simulink model "finalpro"  (R2021a)
settings: Solver=FixedStepAuto  StartTime=0.0  StopTime=25  FixedStep=0.001  RelTol=1e-3
libraries: neural x8, pid_lib x4, fuzblock x1
settings Model: Creator=User  LastModifiedBy=User

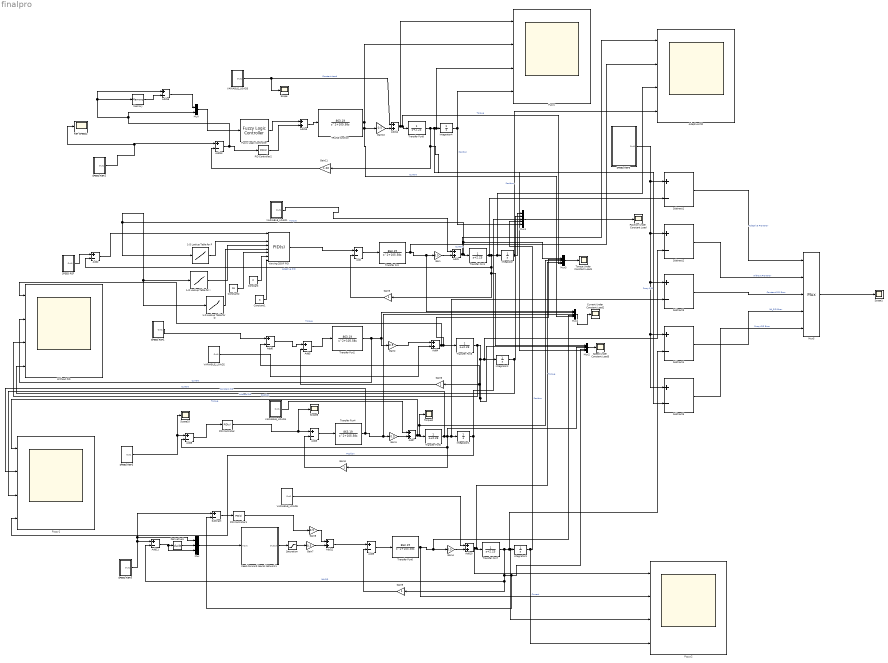
== system finalpro ==
  1-D Lookup Table for D : Lookup_n-D  NumberOfTableDimensions=1  BreakpointsForDimension1=[-5, -4.5, -4, -3.5, -3, -2.5, -2, -1.5, -1, -0.5, 0, 0.5, 1, 1.5, 2, 2.5, 3, 3.5, 4, 4.5, 5, 5.5, 6, 6.5, 7, 7.5, 8, 8.5, 9, 9.5, 10]  Table=[0.1, 0.1, 0.1, 0.1, 0.1, 0.1, 0.1, 0.1, 0.1, 0.1, 0.1, 0.1, 0.1, 0.1, 0.1, 0.1, 0.1, 0.1, 0.1, 0.1, 0.1, 0.1, 0.1, 0.1, 0.1, 0.1, 0.1, 0.1, 0.1, 0.1, 0.1]  InterpMethod=Linear Lagrange  InternalRulePriority=Speed  RndMeth=Simplest  InputSameDT=on
  1-D Lookup Table for I : Lookup_n-D  NumberOfTableDimensions=1  BreakpointsForDimension1=[-5, -4.5, -4, -3.5, -3, -2.5, -2, -1.5, -1, -0.5, 0, 0.5, 1, 1.5, 2, 2.5, 3, 3.5, 4, 4.5, 5, 5.5, 6, 6.5, 7, 7.5, 8, 8.5, 9, 9.5, 10]  Table=[2.0, 2.0, 2.0, 2.0, 2.0, 0.1, 0.1, 0.1, 2.0, 0.5, 0.5, 0.5, 0.5, 0.5, 0.5, 2.5, 2.5, 2.5, 2.0, 2.0, 2.0, 2.0, 0.5, 0.5, 0.5, 2.0, 2.0, 2.0, 2.0, 2.0, 2.0]  InternalRulePriority=Speed  RndMeth=Simplest  InputSameDT=on
  1-D Lookup Table for P : Lookup_n-D  NumberOfTableDimensions=1  BreakpointsForDimension1=[-5, -4.5, -4, -3.5, -3, -2.5, -2, -1.5, -1, -0.5, 0, 0.5, 1, 1.5, 2, 2.5, 3, 3.5, 4, 4.5, 5, 5.5, 6, 6.5, 7, 7.5, 8, 8.5, 9, 9.5, 10]  Table=[2.0, 2.0, 0.5, 0.05, 0.05, 0.5, 0.1, 1, 1.5, 1.5, 1.5, 1.5, 2.0, 2.0, 2.5, .05, .5, .5, 2.0, 2.0, 2.0, 2.0, 0.5, 0.5, 0.5, 2.0, 2.0, 2.0, 2.0, 2.0, 2.0]  InterpMethod=Linear Lagrange  InternalRulePriority=Speed  RndMeth=Simplest  InputSameDT=on
  Adaptive PID : Scope  NumInputPorts=4
  Add{,2..3,5..6,8..9,11,13,16} (10 alike) : Sum  Inputs=+-
  Add{1,4,7,10,12,14..15} (7 alike) : Sum
  Constant : Constant  Value=2
  Constant1 : Constant  Value=3
  Constant2 : Constant  Value=15
  Current Under Constant Load2 : Scope
  Derivative1 : Derivative
  Feed-Forward Neural Network1 : Subsystem
      mask help: Feed-Forward Neural Network
      mask Display: e = 0.06;c1 = [120 150 230]/255;c2 = ([120 150 230]+0)/383;c3 = ([120 150 230]+128)/383;patch([0 1 1 0],[0 0 1 1],c1);patch([0 1 1 1-e 1-e 0+e],[0 0 1 1-e 0+e 0+e],c2);patch([0 0 1 1-e 0+e 0+e],[0 1 1 1-e 1-e 0+e],c3);plot([0 1 1 0 0],[0 0 1 1 0]);fprintf('NNET');port_label('input',1,' Input');port_label('output',1,'Output ');
  Fuzzy : Scope  NumInputPorts=4
  Fuzzy Logic Controller : fuzblock/Fuzzy Logic  Controller  FIS='DCMotorFLC.fis'  OutputSampleNumber=101  DataType=double  FuzzifiedInputs=off  RuleFiringStrengths=off  RuleOutputs=off  AggregatedOutputs=off  SimulateUsing=Interpreted execution  OutOfRangeInputValueMessage=warning  NoRuleFiredMessage=warning  EmptyOutputFuzzySetMessage=warning
  Fuzzy1 : Scope  NumInputPorts=4
  Fuzzy2 : Scope  NumInputPorts=4
  Gain{,1..2,4,7..8,10} (7 alike) : Gain  Gain=0.5
  Gain11 : Gain  Gain=1.02
  Gain{3,5..6,9} (4 alike) : Gain
  Integrator{,1..4} (5 alike) : Integrator
  MUX : Mux  Inputs=2
  Memory : Memory
  Mux : Mux  Inputs=3
  Mux{1..5} (5 alike) : Mux  Inputs=5
  PID Controller : pid_lib/PID Controller  Controller=PID  Form=Parallel  TimeDomain=Continuous-time  UseExternalTs=off  SampleTime=-1  IntegratorMethod=Forward Euler  FilterMethod=Forward Euler  ControllerParametersSource=internal  P=2  I=2.2  D=0.8  UseFilter=on  N=358.799773599194  TunerSelectOption=Transfer Function Based (PID Tuner App)  InitialConditionSource=internal  InitialConditionForIntegrator=0  InitialConditionForFilter=0  DifferentiatorICPrevScaledInput=0  ExternalReset=none  TrackingMode=off  Kt=1  LimitOutput=off  SatLimitsSource=internal  UpperSaturationLimit=inf  LowerSaturationLimit=-inf  LinearizeAsGain=on  AntiWindupMode=none  Kb=1  POutMin=[]  POutMax=[]  IOutMin=[]  IOutMax=[]  DOutMin=[]  DOutMax=[]  NOutMin=[]  NOutMax=[]  SumOutMin=[]  SumOutMax=[]  SaturationOutMin=[]  SaturationOutMax=[]  PParamMin=[]  PParamMax=[]  IParamMin=[]  IParamMax=[]  DParamMin=[]  DParamMax=[]  NParamMin=[]  NParamMax=[]  KbParamMin=[]  KbParamMax=[]  KtParamMin=[]  KtParamMax=[]  KbOutMin=[]  KbOutMax=[]  KtOutMin=[]  KtOutMax=[]  IntegratorOutMin=[]  IntegratorOutMax=[]  FilterOutMin=[]  FilterOutMax=[]  SumI1OutMin=[]  SumI1OutMax=[]  SumI2OutMin=[]  SumI2OutMax=[]  SumI3OutMin=[]  SumI3OutMax=[]  SumI4OutMin=[]  SumI4OutMax=[]  SumDOutMin=[]  SumDOutMax=[]  DifferentiatorOutMin=[]  DifferentiatorOutMax=[]  FilterDiffOutCoefMin=[]  FilterDiffOutCoefMax=[]  ReciprocalOutMin=[]  ReciprocalOutMax=[]  SumDenOutMin=[]  SumDenOutMax=[]  SumNumOutMin=[]  SumNumOutMax=[]  DivideOutMin=[]  DivideOutMax=[]  UdiffTsProdOutMin=[]  UdiffTsProdOutMax=[]  NTsProdOutMin=[]  NTsProdOutMax=[]  UintegralTsProdOutMin=[]  UintegralTsProdOutMax=[]  UngainTsProdOutMin=[]  UngainTsProdOutMax=[]  IntegratorContinuousStateAttributes=''  IntegratorStateMustResolveToSignalObject=off  IntegratorRTWStateStorageClass=Auto  FilterContinuousStateAttributes=''  FilterStateMustResolveToSignalObject=off  FilterRTWStateStorageClass=Auto  ParallelPVariant=InternalParameters  IdealPVariant=Disabled  IVariant=InternalParameters  DVariant=InternalParameters  IntegratorVariant=Continuous  SatVariant=Disabled  AWVariant=Passthrough  PCopyVariant=Disabled  TRVariant=Disabled  FdbkBlocksVariant=Forward  IdealPFdbkVariant=Disabled  SatFdbkVariant=Disabled  DerivativeFilterVariant=ContFilter  NVariant=InternalParameters  NCopyVariant=Disabled  FilterICVariant=InternalICsFilter  IntegratorICVariant=InternalICs  ExternalResetVariant=Disabled  TRSumVariant=Passthrough  SumFdbkVariant=Disabled  SumVariant=Sum_PID  TsampFilterVariant=InternalTs  TsampNgainVariant=Passthrough  TsampIntegralVariant=Passthrough  ExternalSaturationOutDataTypeStr=Inherit: Same as second input
  PID Controller1 : pid_lib/PID Controller  Controller=PID  Form=Parallel  TimeDomain=Continuous-time  UseExternalTs=off  SampleTime=-1  IntegratorMethod=Forward Euler  FilterMethod=Forward Euler  ControllerParametersSource=internal  P=2  I=2.2  D=0.8  UseFilter=on  N=358.799773599194  TunerSelectOption=Transfer Function Based (PID Tuner App)  InitialConditionSource=internal  InitialConditionForIntegrator=0  InitialConditionForFilter=0  DifferentiatorICPrevScaledInput=0  ExternalReset=none  TrackingMode=off  Kt=1  LimitOutput=off  SatLimitsSource=internal  UpperSaturationLimit=inf  LowerSaturationLimit=-inf  LinearizeAsGain=on  AntiWindupMode=none  Kb=1  POutMin=[]  POutMax=[]  IOutMin=[]  IOutMax=[]  DOutMin=[]  DOutMax=[]  NOutMin=[]  NOutMax=[]  SumOutMin=[]  SumOutMax=[]  SaturationOutMin=[]  SaturationOutMax=[]  PParamMin=[]  PParamMax=[]  IParamMin=[]  IParamMax=[]  DParamMin=[]  DParamMax=[]  NParamMin=[]  NParamMax=[]  KbParamMin=[]  KbParamMax=[]  KtParamMin=[]  KtParamMax=[]  KbOutMin=[]  KbOutMax=[]  KtOutMin=[]  KtOutMax=[]  IntegratorOutMin=[]  IntegratorOutMax=[]  FilterOutMin=[]  FilterOutMax=[]  SumI1OutMin=[]  SumI1OutMax=[]  SumI2OutMin=[]  SumI2OutMax=[]  SumI3OutMin=[]  SumI3OutMax=[]  SumI4OutMin=[]  SumI4OutMax=[]  SumDOutMin=[]  SumDOutMax=[]  DifferentiatorOutMin=[]  DifferentiatorOutMax=[]  FilterDiffOutCoefMin=[]  FilterDiffOutCoefMax=[]  ReciprocalOutMin=[]  ReciprocalOutMax=[]  SumDenOutMin=[]  SumDenOutMax=[]  SumNumOutMin=[]  SumNumOutMax=[]  DivideOutMin=[]  DivideOutMax=[]  UdiffTsProdOutMin=[]  UdiffTsProdOutMax=[]  NTsProdOutMin=[]  NTsProdOutMax=[]  UintegralTsProdOutMin=[]  UintegralTsProdOutMax=[]  UngainTsProdOutMin=[]  UngainTsProdOutMax=[]  IntegratorContinuousStateAttributes=''  IntegratorStateMustResolveToSignalObject=off  IntegratorRTWStateStorageClass=Auto  FilterContinuousStateAttributes=''  FilterStateMustResolveToSignalObject=off  FilterRTWStateStorageClass=Auto  ParallelPVariant=InternalParameters  IdealPVariant=Disabled  IVariant=InternalParameters  DVariant=InternalParameters  IntegratorVariant=Continuous  SatVariant=Disabled  AWVariant=Passthrough  PCopyVariant=Disabled  TRVariant=Disabled  FdbkBlocksVariant=Forward  IdealPFdbkVariant=Disabled  SatFdbkVariant=Disabled  DerivativeFilterVariant=ContFilter  NVariant=InternalParameters  NCopyVariant=Disabled  FilterICVariant=InternalICsFilter  IntegratorICVariant=InternalICs  ExternalResetVariant=Disabled  TRSumVariant=Passthrough  SumFdbkVariant=Disabled  SumVariant=Sum_PID  TsampFilterVariant=InternalTs  TsampNgainVariant=Passthrough  TsampIntegralVariant=Passthrough  ExternalSaturationOutDataTypeStr=Inherit: Same as second input
  PID Controller2 : pid_lib/PID Controller  Controller=PID  Form=Parallel  TimeDomain=Continuous-time  UseExternalTs=off  SampleTime=-1  IntegratorMethod=Forward Euler  FilterMethod=Forward Euler  ControllerParametersSource=internal  P=1.8  I=0.6  D=0.5  UseFilter=on  N=100  TunerSelectOption=Transfer Function Based (PID Tuner App)  InitialConditionSource=internal  InitialConditionForIntegrator=0  InitialConditionForFilter=0  DifferentiatorICPrevScaledInput=0  ExternalReset=none  TrackingMode=off  Kt=1  LimitOutput=off  SatLimitsSource=internal  UpperSaturationLimit=inf  LowerSaturationLimit=-inf  LinearizeAsGain=on  AntiWindupMode=none  Kb=1  POutMin=[]  POutMax=[]  IOutMin=[]  IOutMax=[]  DOutMin=[]  DOutMax=[]  NOutMin=[]  NOutMax=[]  SumOutMin=[]  SumOutMax=[]  SaturationOutMin=[]  SaturationOutMax=[]  PParamMin=[]  PParamMax=[]  IParamMin=[]  IParamMax=[]  DParamMin=[]  DParamMax=[]  NParamMin=[]  NParamMax=[]  KbParamMin=[]  KbParamMax=[]  KtParamMin=[]  KtParamMax=[]  KbOutMin=[]  KbOutMax=[]  KtOutMin=[]  KtOutMax=[]  IntegratorOutMin=[]  IntegratorOutMax=[]  FilterOutMin=[]  FilterOutMax=[]  SumI1OutMin=[]  SumI1OutMax=[]  SumI2OutMin=[]  SumI2OutMax=[]  SumI3OutMin=[]  SumI3OutMax=[]  SumI4OutMin=[]  SumI4OutMax=[]  SumDOutMin=[]  SumDOutMax=[]  DifferentiatorOutMin=[]  DifferentiatorOutMax=[]  FilterDiffOutCoefMin=[]  FilterDiffOutCoefMax=[]  ReciprocalOutMin=[]  ReciprocalOutMax=[]  SumDenOutMin=[]  SumDenOutMax=[]  SumNumOutMin=[]  SumNumOutMax=[]  DivideOutMin=[]  DivideOutMax=[]  UdiffTsProdOutMin=[]  UdiffTsProdOutMax=[]  NTsProdOutMin=[]  NTsProdOutMax=[]  UintegralTsProdOutMin=[]  UintegralTsProdOutMax=[]  UngainTsProdOutMin=[]  UngainTsProdOutMax=[]  IntegratorContinuousStateAttributes=''  IntegratorStateMustResolveToSignalObject=off  IntegratorRTWStateStorageClass=Auto  FilterContinuousStateAttributes=''  FilterStateMustResolveToSignalObject=off  FilterRTWStateStorageClass=Auto  ParallelPVariant=InternalParameters  IdealPVariant=Disabled  IVariant=InternalParameters  DVariant=InternalParameters  IntegratorVariant=Continuous  SatVariant=Disabled  AWVariant=Passthrough  PCopyVariant=Disabled  TRVariant=Disabled  FdbkBlocksVariant=Forward  IdealPFdbkVariant=Disabled  SatFdbkVariant=Disabled  DerivativeFilterVariant=ContFilter  NVariant=InternalParameters  NCopyVariant=Disabled  FilterICVariant=InternalICsFilter  IntegratorICVariant=InternalICs  ExternalResetVariant=Disabled  TRSumVariant=Passthrough  SumFdbkVariant=Disabled  SumVariant=Sum_PID  TsampFilterVariant=InternalTs  TsampNgainVariant=Passthrough  TsampIntegralVariant=Passthrough  ExternalSaturationOutDataTypeStr=Inherit: Same as second input
  Position Under Constant Load : Scope
  REF SPEED2 : Scope
  SPEED REF : Subsystem
  SPEED REF1 : Subsystem
  SPEED REF2 : Subsystem
  SPEED REF3 : Subsystem
  SPEED REF4 : Subsystem
  SPEED REF5 : Subsystem
  Saturation : Saturate  UpperLimit=1  LowerLimit=-1
  Scope{,1,8,10} (4 alike) : Scope
  Speed Under Constant Load3 : Scope
  Subtract{,1..5} (6 alike) : Sum  Inputs=+-
  TRANS function : TransferFcn  Numerator=[863.19]  Denominator=[1 105.58 0]
  Torque Under Constant Load1 : Scope
  Torque2 : Scope
  Transfer Fcn{,2,4,6} (4 alike) : TransferFcn  Numerator=[863.19]  Denominator=[1 105.58 0]
  Transfer Fcn{1,3,5,7..8} (5 alike) : TransferFcn  Denominator=[1 2.23]
  VARIABLE_LOAD1 : Subsystem
  VARIABLE_LOAD2 : Subsystem
  VARIABLE_LOAD3 : Subsystem
  VARIABLE_LOAD4 : Subsystem
  VARIABLE_LOAD5 : Subsystem
  Varying 2DOF PID : pid_lib/PID Controller (2DOF)  Controller=PID  Form=Parallel  TimeDomain=Continuous-time  UseExternalTs=off  SampleTime=-1  IntegratorMethod=Forward Euler  FilterMethod=Forward Euler  ControllerParametersSource=external  P=1  I=1  D=0  UseFilter=on  N=100  b=1  c=1  TunerSelectOption=Transfer Function Based (PID Tuner App)  InitialConditionSource=internal  InitialConditionForIntegrator=0  InitialConditionForFilter=0  DifferentiatorICPrevScaledInput=0  ExternalReset=none  TrackingMode=off  Kt=1  LimitOutput=off  SatLimitsSource=internal  UpperSaturationLimit=inf  LowerSaturationLimit=-inf  LinearizeAsGain=on  AntiWindupMode=none  Kb=1  POutMin=[]  POutMax=[]  IOutMin=[]  IOutMax=[]  DOutMin=[]  DOutMax=[]  NOutMin=[]  NOutMax=[]  bOutMin=[]  bOutMax=[]  cOutMin=[]  cOutMax=[]  SumOutMin=[]  SumOutMax=[]  SaturationOutMin=[]  SaturationOutMax=[]  PParamMin=[]  PParamMax=[]  IParamMin=[]  IParamMax=[]  DParamMin=[]  DParamMax=[]  NParamMin=[]  NParamMax=[]  bParamMin=[]  bParamMax=[]  cParamMin=[]  cParamMax=[]  KbParamMin=[]  KbParamMax=[]  KtParamMin=[]  KtParamMax=[]  KbOutMin=[]  KbOutMax=[]  KtOutMin=[]  KtOutMax=[]  IntegratorOutMin=[]  IntegratorOutMax=[]  FilterOutMin=[]  FilterOutMax=[]  SumI1OutMin=[]  SumI1OutMax=[]  SumI2OutMin=[]  SumI2OutMax=[]  SumI3OutMin=[]  SumI3OutMax=[]  SumI4OutMin=[]  SumI4OutMax=[]  SumDOutMin=[]  SumDOutMax=[]  Sum1OutMin=[]  Sum1OutMax=[]  Sum2OutMin=[]  Sum2OutMax=[]  Sum3OutMin=[]  Sum3OutMax=[]  DifferentiatorOutMin=[]  DifferentiatorOutMax=[]  FilterDiffOutCoefMin=[]  FilterDiffOutCoefMax=[]  ReciprocalOutMin=[]  ReciprocalOutMax=[]  SumDenOutMin=[]  SumDenOutMax=[]  SumNumOutMin=[]  SumNumOutMax=[]  DivideOutMin=[]  DivideOutMax=[]  UdiffTsProdOutMin=[]  UdiffTsProdOutMax=[]  NTsProdOutMin=[]  NTsProdOutMax=[]  UintegralTsProdOutMin=[]  UintegralTsProdOutMax=[]  UngainTsProdOutMin=[]  UngainTsProdOutMax=[]  IntegratorContinuousStateAttributes=''  IntegratorStateMustResolveToSignalObject=off  IntegratorRTWStateStorageClass=Auto  FilterContinuousStateAttributes=''  FilterStateMustResolveToSignalObject=off  FilterRTWStateStorageClass=Auto  ParallelPVariant=ExternalParameters  IdealPVariant=Disabled  IVariant=ExternalParameters  DVariant=ExternalParameters  bVariant=ExternalParameters  cVariant=ExternalParameters  IntegratorVariant=Continuous  SatVariant=Disabled  AWVariant=Passthrough  PCopyVariant=Disabled  TRVariant=Disabled  FdbkBlocksVariant=Forward  IdealPFdbkVariant=Disabled  SatFdbkVariant=Disabled  DerivativeFilterVariant=ContFilter  NVariant=ExternalParameters  NCopyVariant=Disabled  FilterICVariant=InternalICsFilter  IntegratorICVariant=InternalICs  ExternalResetVariant=Disabled  TRSumVariant=Passthrough  SumFdbkVariant=Disabled  SumVariant=Sum_PID  TsampFilterVariant=InternalTs  TsampNgainVariant=Passthrough  TsampIntegralVariant=Passthrough  ExternalSaturationOutDataTypeStr=Inherit: Same as second input
      settings: SourceProductBaseCode=SL
  Without PID : Scope  NumInputPorts=4
  wires:
  Transfer Fcn8/1 -> Gain11/1, Mux2/5, Subtract5/2, Fuzzy/3, Integrator4/1  "Fuzzy-PID"
  MUX/1 -> Fuzzy Logic Controller/1
  Fuzzy Logic Controller/1 -> Add15/1
  Gain10/1 -> Add14/2
  Add16/1 -> MUX/1
  TRANS function/1 -> Fuzzy/2, Mux4/5, Gain10/1  "Current"
  Add14/1 -> Fuzzy/1, Mux3/5, Transfer Fcn8/1  "Torque"
  Add15/1 -> TRANS function/1
  SPEED REF4/1(Out1) -> Add13/1, REF SPEED2/1
  Add13/1 -> MUX/2, Memory/1, Add16/1, PID Controller2/1
  Memory/1 -> Add16/2
  PID Controller2/1 -> Add15/2
  Mux/1 -> Feed-Forward Neural Network1/1(Input)
  Add9/1 -> Transfer Fcn6/1
  Transfer Fcn7/1 -> Gain9/1, Add11/2, Subtract/2, Mux2/4, Subtract4/2, Fuzzy2/3, Integrator3/1  "NN-PID"
  Gain9/1 -> Add9/2
  Subtract/1 -> PID Controller1/1
  Gain4/1 -> Add10/2
  Gain2/1 -> Add4/1
  Add8/1 -> PID Controller/1
  VARIABLE_LOAD2/1(Out1) -> Add4/2
  Gain/1 -> Add1/2
  Add11/1 -> Mux/3, Derivative1/1
  SPEED REF3/1(Out1) -> Subtract/1, Mux/1, Add11/1
  Add1/1 -> Adaptive PID/1, 1-D Lookup Table for D/1, 1-D Lookup Table for I/1, 1-D Lookup Table for P/1, Mux3/1, Transfer Fcn1/1  "Torque"
  Transfer Fcn6/1 -> Fuzzy2/2, Mux4/4, Gain4/1  "Current"
  Gain8/1 -> Add12/1
  Mux4/1 -> Current Under Constant Load2/1
  Add12/1 -> Add9/1
  Gain5/1 -> Add/2
  Add10/1 -> Fuzzy2/1, Mux3/4, Transfer Fcn7/1  "Torque"
  Add3/1 -> Transfer Fcn4/1
  Add7/1 -> Fuzzy1/1, Mux3/3, Torque2/1, Transfer Fcn5/1  "Torque"
  Saturation/1 -> Gain7/1
  SPEED REF2/1(Out1) -> Scope10/1, Add8/1
  Varying 2DOF PID/1 -> Add/1
  Add4/1 -> Without PID/1, Mux3/2, Transfer Fcn3/1  "Torque"
  Gain7/1 -> Add12/2
  SPEED REF1/1(Out1) -> Add6/1
  Gain6/1 -> Add5/2
  Gain11/1 -> Add13/2
  Add6/1 -> Add5/1
  Transfer Fcn1/1 -> Subtract1/2, Gain5/1, Mux2/1, Add2/2, Adaptive PID/3, Integrator/1  "Adaptive PID"
  Transfer Fcn2/1 -> Without PID/2, Mux4/2, Gain2/1  "Current"
  Gain1/1 -> Add7/2
  Add2/1 -> Varying 2DOF PID/1
  Constant1/1 -> Varying 2DOF PID/8
  Transfer Fcn4/1 -> Fuzzy1/2, Mux4/3, Gain1/1  "Current"
  Transfer Fcn/1 -> Adaptive PID/2, Mux4/1, Gain/1  "Current"
  Mux1/1 -> Position Under Constant Load/1
  Mux2/1 -> Speed Under Constant Load3/1
  Integrator1/1 -> Mux1/3, Fuzzy1/4  "Position"
  Add/1 -> Transfer Fcn/1
  Constant2/1 -> Varying 2DOF PID/6
  Constant/1 -> Varying 2DOF PID/7
  1-D Lookup Table for P/1 -> Varying 2DOF PID/3
  Derivative1/1 -> Mux/2
  SPEED REF/1(Out1) -> Add2/1
  VARIABLE_LOAD3/1(Out1) -> Scope/1, Add14/1  "Constant Load"
  Transfer Fcn3/1 -> Without PID/3, Mux2/2, Add6/2, Gain6/1, Subtract2/2, Integrator2/1  "Without PID"
  Integrator/1 -> Adaptive PID/4, Mux1/1  "Position"
  VARIABLE_LOAD4/1(Out1) -> Add7/1
  PID Controller1/1 -> Gain8/1
  Gain3/1 -> Add3/2
  1-D Lookup Table for I/1 -> Varying 2DOF PID/4
  Add5/1 -> Transfer Fcn2/1
  Integrator2/1 -> Without PID/4, Mux1/2  "Position"
  PID Controller/1 -> Scope8/1, Add3/1
  VARIABLE_LOAD1/1(Out1) -> Add1/1
  1-D Lookup Table for D/1 -> Varying 2DOF PID/5
  Feed-Forward Neural Network1/1(Output) -> Saturation/1
  VARIABLE_LOAD5/1(Out1) -> Add10/1
  Transfer Fcn5/1 -> Fuzzy1/3, Mux2/3, Gain3/1, Add8/2, Subtract3/2, Integrator1/1  "Constant PID"
  SPEED REF5/1(Out1) -> Subtract2/1, Subtract5/1, Subtract4/1, Subtract3/1, Subtract1/1
  Integrator3/1 -> Fuzzy2/4, Mux1/4  "Position"
  Integrator4/1 -> Mux1/5, Fuzzy/4  "Position"
  Mux3/1 -> Torque Under Constant Load1/1
  Subtract1/1 -> Mux5/1  "Adaptive PID Error"
  Subtract2/1 -> Mux5/2  "Without PID Error"
  Subtract3/1 -> Mux5/3  "Constant PID Error"
  Subtract4/1 -> Mux5/4  "NN_PID Error"
  Subtract5/1 -> Mux5/5  "Fuzzy-PID Error"
  Mux5/1 -> Scope1/1

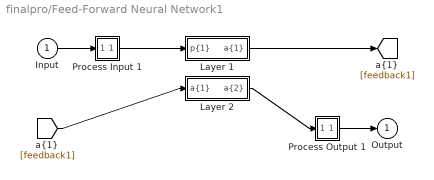
== system finalpro/Feed-Forward Neural Network1 ==
  Input : Inport  PortDimensions=3  SampleTime=0.01
      mask Display: e = 0.06;c1 = [120 230 180]/255;c2 = ([120 230 180]+0)/(256+128);c3 = ([120 230 180]+128)/(256+128);patch([0 1 1 0],[0 0 1 1],c1);patch([0 1 1 1-e 1-e 0+e],[0 0 1 1-e 0+e 0+e],c2);patch([0 0 1 1-e 0+e 0+e],[0 1 1 1-e 1-e 0+e],c3);plot([0 1 1 0 0],[0 0 1 1 0]);
  Layer 1 : Subsystem
      mask Display: e = 0.06;c1 = [120 150 230]/255;c2 = ([120 150 230]+0)/383;c3 = ([120 150 230]+128)/383;patch([0 1 1 0],[0 0 1 1],c1);patch([0 1 1 1-e 1-e 0+e],[0 0 1 1-e 0+e 0+e],c2);patch([0 0 1 1-e 0+e 0+e],[0 1 1 1-e 1-e 0+e],c3);plot([0 1 1 0 0],[0 0 1 1 0]);
  Layer 2 : Subsystem
      mask Display: e = 0.06;c1 = [120 150 230]/255;c2 = ([120 150 230]+0)/383;c3 = ([120 150 230]+128)/383;patch([0 1 1 0],[0 0 1 1],c1);patch([0 1 1 1-e 1-e 0+e],[0 0 1 1-e 0+e 0+e],c2);patch([0 0 1 1-e 0+e 0+e],[0 1 1 1-e 1-e 0+e],c3);plot([0 1 1 0 0],[0 0 1 1 0]);
  Process Input 1 : Subsystem
      mask Display: e = 0.06;c1 = [120 150 230]/255;c2 = ([120 150 230]+0)/383;c3 = ([120 150 230]+128)/383;patch([0 1 1 0],[0 0 1 1],c1);patch([0 1 1 1-e 1-e 0+e],[0 0 1 1-e 0+e 0+e],c2);patch([0 0 1 1-e 0+e 0+e],[0 1 1 1-e 1-e 0+e],c3);plot([0 1 1 0 0],[0 0 1 1 0]);
  Process Output 1 : Subsystem
      mask Display: e = 0.06;c1 = [120 150 230]/255;c2 = ([120 150 230]+0)/383;c3 = ([120 150 230]+128)/383;patch([0 1 1 0],[0 0 1 1],c1);patch([0 1 1 1-e 1-e 0+e],[0 0 1 1-e 0+e 0+e],c2);patch([0 0 1 1-e 0+e 0+e],[0 1 1 1-e 1-e 0+e],c3);plot([0 1 1 0 0],[0 0 1 1 0]);
  Output : Outport  InitialOutput=0
      mask Display: e = 0.06;c1 = [120 230 180]/255;c2 = ([120 230 180]+0)/(256+128);c3 = ([120 230 180]+128)/(256+128);patch([0 1 1 0],[0 0 1 1],c1);patch([0 1 1 1-e 1-e 0+e],[0 0 1 1-e 0+e 0+e],c2);patch([0 0 1 1-e 0+e 0+e],[0 1 1 1-e 1-e 0+e],c3);plot([0 1 1 0 0],[0 0 1 1 0]);
  wires:
  Layer 2/1("a{2}") -> Process Output 1/1(a)
  [feedback1] -> Layer 2/1("a{1} ")
  Layer 1/1("a{1}") -> [feedback1]
  Process Input 1/1(p) -> Layer 1/1("p{1}")
  Process Output 1/1(y) -> Output/1
  Input/1 -> Process Input 1/1(x)

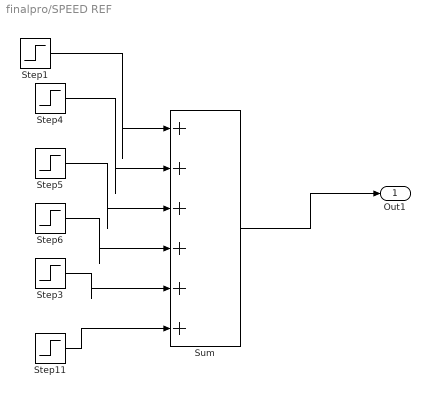
== system finalpro/SPEED REF ==
  Step1 : Step  Time=0  Before=2  After=0  SampleTime=0
  Step11 : Step  Time=0  SampleTime=0
  Step3 : Step  Time=20  SampleTime=0
  Step4 : Step  Time=5  Before=1  After=0  SampleTime=0
  Step5 : Step  Time=10  Before=0  After=-1  SampleTime=0
  Step6 : Step  Time=15  Before=-1  After=0  SampleTime=0
  Sum : Sum  Inputs=|++++++
  Out1 : Outport
  wires:
  Step5/1 -> Sum/3
  Step3/1 -> Sum/5
  Step11/1 -> Sum/6
  Step1/1 -> Sum/1
  Sum/1 -> Out1/1
  Step4/1 -> Sum/2
  Step6/1 -> Sum/4

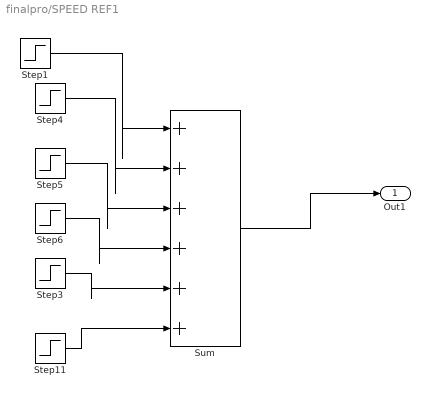
== system finalpro/SPEED REF1 ==
  Step1 : Step  Time=0  Before=2  After=0  SampleTime=0
  Step11 : Step  Time=0  SampleTime=0
  Step3 : Step  Time=20  SampleTime=0
  Step4 : Step  Time=5  Before=1  After=0  SampleTime=0
  Step5 : Step  Time=10  Before=0  After=-1  SampleTime=0
  Step6 : Step  Time=15  Before=-1  After=0  SampleTime=0
  Sum : Sum  Inputs=|++++++
  Out1 : Outport
  wires:
  Step5/1 -> Sum/3
  Step3/1 -> Sum/5
  Step11/1 -> Sum/6
  Step1/1 -> Sum/1
  Sum/1 -> Out1/1
  Step4/1 -> Sum/2
  Step6/1 -> Sum/4

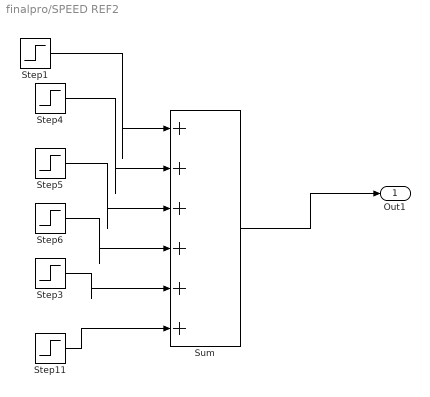
== system finalpro/SPEED REF2 ==
  Step1 : Step  Time=0  Before=2  After=0  SampleTime=0
  Step11 : Step  Time=0  SampleTime=0
  Step3 : Step  Time=20  SampleTime=0
  Step4 : Step  Time=5  Before=1  After=0  SampleTime=0
  Step5 : Step  Time=10  Before=0  After=-1  SampleTime=0
  Step6 : Step  Time=15  Before=-1  After=0  SampleTime=0
  Sum : Sum  Inputs=|++++++
  Out1 : Outport
  wires:
  Step5/1 -> Sum/3
  Step3/1 -> Sum/5
  Step11/1 -> Sum/6
  Step1/1 -> Sum/1
  Sum/1 -> Out1/1
  Step4/1 -> Sum/2
  Step6/1 -> Sum/4

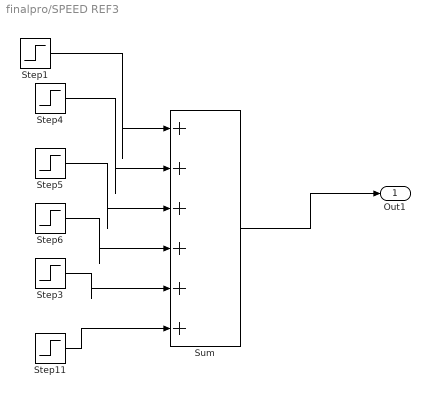
== system finalpro/SPEED REF3 ==
  Step1 : Step  Time=0  Before=2  After=0  SampleTime=0
  Step11 : Step  Time=0  SampleTime=0
  Step3 : Step  Time=20  SampleTime=0
  Step4 : Step  Time=5  Before=1  After=0  SampleTime=0
  Step5 : Step  Time=10  Before=0  After=-1  SampleTime=0
  Step6 : Step  Time=15  Before=-1  After=0  SampleTime=0
  Sum : Sum  Inputs=|++++++
  Out1 : Outport
  wires:
  Step5/1 -> Sum/3
  Step3/1 -> Sum/5
  Step11/1 -> Sum/6
  Step1/1 -> Sum/1
  Sum/1 -> Out1/1
  Step4/1 -> Sum/2
  Step6/1 -> Sum/4

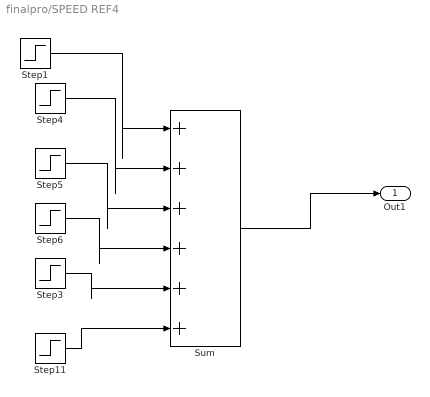
== system finalpro/SPEED REF4 ==
  Step1 : Step  Time=0  Before=2  After=0  SampleTime=0
  Step11 : Step  Time=0  SampleTime=0
  Step3 : Step  Time=20  SampleTime=0
  Step4 : Step  Time=5  Before=1  After=0  SampleTime=0
  Step5 : Step  Time=10  Before=0  After=-1  SampleTime=0
  Step6 : Step  Time=15  Before=-1  After=0  SampleTime=0
  Sum : Sum  Inputs=|++++++
  Out1 : Outport
  wires:
  Step5/1 -> Sum/3
  Step3/1 -> Sum/5
  Step11/1 -> Sum/6
  Step1/1 -> Sum/1
  Sum/1 -> Out1/1
  Step4/1 -> Sum/2
  Step6/1 -> Sum/4

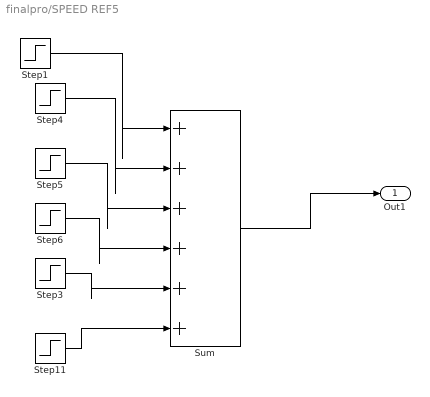
== system finalpro/SPEED REF5 ==
  Step1 : Step  Time=0  Before=2  After=0  SampleTime=0
  Step11 : Step  Time=0  SampleTime=0
  Step3 : Step  Time=20  SampleTime=0
  Step4 : Step  Time=5  Before=1  After=0  SampleTime=0
  Step5 : Step  Time=10  Before=0  After=-1  SampleTime=0
  Step6 : Step  Time=15  Before=-1  After=0  SampleTime=0
  Sum : Sum  Inputs=|++++++
  Out1 : Outport
  wires:
  Step5/1 -> Sum/3
  Step3/1 -> Sum/5
  Step11/1 -> Sum/6
  Step1/1 -> Sum/1
  Sum/1 -> Out1/1
  Step4/1 -> Sum/2
  Step6/1 -> Sum/4

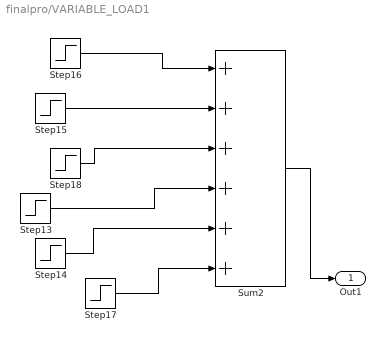
== system finalpro/VARIABLE_LOAD1 ==
  Step13 : Step  Time=10  Before=0  After=0  SampleTime=0
  Step14 : Step  Time=15  After=0  SampleTime=0
  Step15 : Step  Time=0  Before=1  After=0  SampleTime=0
  Step16 : Step  Time=0  After=3  SampleTime=0
  Step17 : Step  Time=20  Before=2  SampleTime=0
  Step18 : Step  Time=5  Before=1  After=0  SampleTime=0
  Sum2 : Sum  Inputs=++++++
  Out1 : Outport
  wires:
  Step18/1 -> Sum2/3
  Step16/1 -> Sum2/1
  Step14/1 -> Sum2/5
  Step15/1 -> Sum2/2
  Step17/1 -> Sum2/6
  Step13/1 -> Sum2/4
  Sum2/1 -> Out1/1

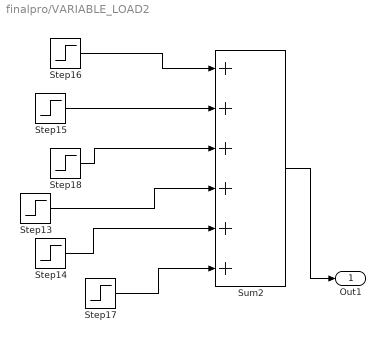
== system finalpro/VARIABLE_LOAD2 ==
  Step13 : Step  Time=10  Before=0  After=0  SampleTime=0
  Step14 : Step  Time=15  After=0  SampleTime=0
  Step15 : Step  Time=0  Before=1  After=0  SampleTime=0
  Step16 : Step  Time=0  After=3  SampleTime=0
  Step17 : Step  Time=20  Before=2  SampleTime=0
  Step18 : Step  Time=5  Before=1  After=0  SampleTime=0
  Sum2 : Sum  Inputs=++++++
  Out1 : Outport
  wires:
  Step18/1 -> Sum2/3
  Step16/1 -> Sum2/1
  Step14/1 -> Sum2/5
  Step15/1 -> Sum2/2
  Step17/1 -> Sum2/6
  Step13/1 -> Sum2/4
  Sum2/1 -> Out1/1

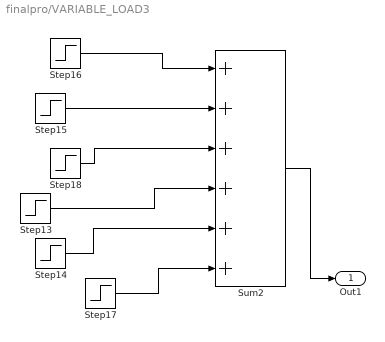
== system finalpro/VARIABLE_LOAD3 ==
  Step13 : Step  Time=10  Before=0  After=0  SampleTime=0
  Step14 : Step  Time=15  After=0  SampleTime=0
  Step15 : Step  Time=0  Before=1  After=0  SampleTime=0
  Step16 : Step  Time=0  After=3  SampleTime=0
  Step17 : Step  Time=20  Before=2  SampleTime=0
  Step18 : Step  Time=5  Before=1  After=0  SampleTime=0
  Sum2 : Sum  Inputs=++++++
  Out1 : Outport
  wires:
  Step18/1 -> Sum2/3
  Step16/1 -> Sum2/1
  Step14/1 -> Sum2/5
  Step15/1 -> Sum2/2
  Step17/1 -> Sum2/6
  Step13/1 -> Sum2/4
  Sum2/1 -> Out1/1

== system finalpro/VARIABLE_LOAD4 ==
  Step13 : Step  Time=10  Before=0  After=0  SampleTime=0
  Step14 : Step  Time=15  After=0  SampleTime=0
  Step15 : Step  Time=0  Before=1  After=0  SampleTime=0
  Step16 : Step  Time=0  After=3  SampleTime=0
  Step17 : Step  Time=20  Before=2  SampleTime=0
  Step18 : Step  Time=5  Before=1  After=0  SampleTime=0
  Sum2 : Sum  Inputs=++++++
  Out1 : Outport
  wires:
  Step18/1 -> Sum2/3
  Step16/1 -> Sum2/1
  Step14/1 -> Sum2/5
  Step15/1 -> Sum2/2
  Step17/1 -> Sum2/6
  Step13/1 -> Sum2/4
  Sum2/1 -> Out1/1

== system finalpro/VARIABLE_LOAD5 ==
  Step13 : Step  Time=10  Before=0  After=0  SampleTime=0
  Step14 : Step  Time=15  After=0  SampleTime=0
  Step15 : Step  Time=0  Before=1  After=0  SampleTime=0
  Step16 : Step  Time=0  After=3  SampleTime=0
  Step17 : Step  Time=20  Before=2  SampleTime=0
  Step18 : Step  Time=5  Before=1  After=0  SampleTime=0
  Sum2 : Sum  Inputs=++++++
  Out1 : Outport
  wires:
  Step18/1 -> Sum2/3
  Step16/1 -> Sum2/1
  Step14/1 -> Sum2/5
  Step15/1 -> Sum2/2
  Step17/1 -> Sum2/6
  Step13/1 -> Sum2/4
  Sum2/1 -> Out1/1

== system finalpro/Feed-Forward Neural Network1/Layer 1 ==
  "p{1}" : Inport  PortDimensions=3  SampleTime=0.01
      mask Display: e = 0.06;c1 = [120 230 180]/255;c2 = ([120 230 180]+0)/(256+128);c3 = ([120 230 180]+128)/(256+128);patch([0 1 1 0],[0 0 1 1],c1);patch([0 1 1 1-e 1-e 0+e],[0 0 1 1-e 0+e 0+e],c2);patch([0 0 1 1-e 0+e 0+e],[0 1 1 1-e 1-e 0+e],c3);plot([0 1 1 0 0],[0 0 1 1 0]);
  Delays 1 : Subsystem
      mask Display: e = 0.06;c1 = [120 150 230]/255;c2 = ([120 150 230]+0)/383;c3 = ([120 150 230]+128)/383;patch([0 1 1 0],[0 0 1 1],c1);patch([0 1 1 1-e 1-e 0+e],[0 0 1 1-e 0+e 0+e],c2);patch([0 0 1 1-e 0+e 0+e],[0 1 1 1-e 1-e 0+e],c3);plot([0 1 1 0 0],[0 0 1 1 0]);disp('0');
  "IW{1,1}" : Subsystem
      mask Display: e = 0.06;c1 = [120 150 230]/255;c2 = ([120 150 230]+0)/383;c3 = ([120 150 230]+128)/383;patch([0 1 1 0],[0 0 1 1],c1);patch([0 1 1 1-e 1-e 0+e],[0 0 1 1-e 0+e 0+e],c2);patch([0 0 1 1-e 0+e 0+e],[0 1 1 1-e 1-e 0+e],c3);plot([0 1 1 0 0],[0 0 1 1 0]);disp('W');
  "b{1}" : Constant  Value=[-9.039784028091073508903718902729451656341552734375;0.007088234032908090863356331823297296068631112575531005859375;5.52122914229548999998087310814298689365386962890625]
      mask Display: e = 0.06;c1 = [120 150 230]/255;c2 = ([120 150 230]+0)/383;c3 = ([120 150 230]+128)/383;patch([0 1 1 0],[0 0 1 1],c1);patch([0 1 1 1-e 1-e 0+e],[0 0 1 1-e 0+e 0+e],c2);patch([0 0 1 1-e 0+e 0+e],[0 1 1 1-e 1-e 0+e],c3);plot([0 1 1 0 0],[0 0 1 1 0]);disp('b');
  netsum : Sum  Inputs=2  InputSameDT=on  SaturateOnIntegerOverflow=on  OutDataTypeStr=Inherit: Same as first input
      mask Display: e = 0.06;c1 = [120 150 230]/255;c2 = ([120 150 230]+0)/383;c3 = ([120 150 230]+128)/383;patch([0 1 1 0],[0 0 1 1],c1);patch([0 1 1 1-e 1-e 0+e],[0 0 1 1-e 0+e 0+e],c2);patch([0 0 1 1-e 0+e 0+e],[0 1 1 1-e 1-e 0+e],c3);plot([0 1 1 0 0],[0 0 1 1 0]);disp('+');
  tansig : neural/Transfer Functions/tansig
  "a{1}" : Outport  InitialOutput=[0;0;0]
      mask Display: e = 0.06;c1 = [120 230 180]/255;c2 = ([120 230 180]+0)/(256+128);c3 = ([120 230 180]+128)/(256+128);patch([0 1 1 0],[0 0 1 1],c1);patch([0 1 1 1-e 1-e 0+e],[0 0 1 1-e 0+e 0+e],c2);patch([0 0 1 1-e 0+e 0+e],[0 1 1 1-e 1-e 0+e],c3);plot([0 1 1 0 0],[0 0 1 1 0]);
  wires:
  tansig/1 -> "a{1}"/1
  netsum/1 -> tansig/1
  "b{1}"/1 -> netsum/2
  "IW{1,1}"/1("iz{1,1}") -> netsum/1
  Delays 1/1("pd{1,1}") -> "IW{1,1}"/1("pd{1,1}")
  "p{1}"/1 -> Delays 1/1("p{1}")

== system finalpro/Feed-Forward Neural Network1/Layer 2 ==
  "a{1} " : Inport  PortDimensions=3  SampleTime=0.01
      mask Display: e = 0.06;c1 = [120 230 180]/255;c2 = ([120 230 180]+0)/(256+128);c3 = ([120 230 180]+128)/(256+128);patch([0 1 1 0],[0 0 1 1],c1);patch([0 1 1 1-e 1-e 0+e],[0 0 1 1-e 0+e 0+e],c2);patch([0 0 1 1-e 0+e 0+e],[0 1 1 1-e 1-e 0+e],c3);plot([0 1 1 0 0],[0 0 1 1 0]);
  Delays 1 : Subsystem
      mask Display: e = 0.06;c1 = [120 150 230]/255;c2 = ([120 150 230]+0)/383;c3 = ([120 150 230]+128)/383;patch([0 1 1 0],[0 0 1 1],c1);patch([0 1 1 1-e 1-e 0+e],[0 0 1 1-e 0+e 0+e],c2);patch([0 0 1 1-e 0+e 0+e],[0 1 1 1-e 1-e 0+e],c3);plot([0 1 1 0 0],[0 0 1 1 0]);disp('0');
  "LW{2,1}" : Subsystem
      mask Display: e = 0.06;c1 = [120 150 230]/255;c2 = ([120 150 230]+0)/383;c3 = ([120 150 230]+128)/383;patch([0 1 1 0],[0 0 1 1],c1);patch([0 1 1 1-e 1-e 0+e],[0 0 1 1-e 0+e 0+e],c2);patch([0 0 1 1-e 0+e 0+e],[0 1 1 1-e 1-e 0+e],c3);plot([0 1 1 0 0],[0 0 1 1 0]);disp('W');
  "b{2}" : Constant  Value=0.677985189695716083946308572194539010524749755859375
      mask Display: e = 0.06;c1 = [120 150 230]/255;c2 = ([120 150 230]+0)/383;c3 = ([120 150 230]+128)/383;patch([0 1 1 0],[0 0 1 1],c1);patch([0 1 1 1-e 1-e 0+e],[0 0 1 1-e 0+e 0+e],c2);patch([0 0 1 1-e 0+e 0+e],[0 1 1 1-e 1-e 0+e],c3);plot([0 1 1 0 0],[0 0 1 1 0]);disp('b');
  netsum : Sum  Inputs=2  InputSameDT=on  SaturateOnIntegerOverflow=on  OutDataTypeStr=Inherit: Same as first input
      mask Display: e = 0.06;c1 = [120 150 230]/255;c2 = ([120 150 230]+0)/383;c3 = ([120 150 230]+128)/383;patch([0 1 1 0],[0 0 1 1],c1);patch([0 1 1 1-e 1-e 0+e],[0 0 1 1-e 0+e 0+e],c2);patch([0 0 1 1-e 0+e 0+e],[0 1 1 1-e 1-e 0+e],c3);plot([0 1 1 0 0],[0 0 1 1 0]);disp('+');
  purelin : neural/Transfer Functions/purelin
  "a{2}" : Outport  InitialOutput=0
      mask Display: e = 0.06;c1 = [120 230 180]/255;c2 = ([120 230 180]+0)/(256+128);c3 = ([120 230 180]+128)/(256+128);patch([0 1 1 0],[0 0 1 1],c1);patch([0 1 1 1-e 1-e 0+e],[0 0 1 1-e 0+e 0+e],c2);patch([0 0 1 1-e 0+e 0+e],[0 1 1 1-e 1-e 0+e],c3);plot([0 1 1 0 0],[0 0 1 1 0]);
  wires:
  purelin/1 -> "a{2}"/1
  netsum/1 -> purelin/1
  "b{2}"/1 -> netsum/2
  "LW{2,1}"/1("lz{2,1}") -> netsum/1
  Delays 1/1("pd{2,1}") -> "LW{2,1}"/1("ad{2,1}")
  "a{1} "/1 -> Delays 1/1("p{2}")

== system finalpro/Feed-Forward Neural Network1/Process Input 1 ==
  x : Inport  PortDimensions=3  SampleTime=0.01
      mask Display: e = 0.06;c1 = [120 230 180]/255;c2 = ([120 230 180]+0)/(256+128);c3 = ([120 230 180]+128)/(256+128);patch([0 1 1 0],[0 0 1 1],c1);patch([0 1 1 1-e 1-e 0+e],[0 0 1 1-e 0+e 0+e],c2);patch([0 0 1 1-e 0+e 0+e],[0 1 1 1-e 1-e 0+e],c3);plot([0 1 1 0 0],[0 0 1 1 0]);
  mapminmax : neural/Processing Functions/mapminmax  xmin=[-1.00115474263305981317273563036;-1000.00424736089325961074791849;-1]  xmax=[1.00115727908462170958614478877;1000.00154898429991590091958642;1]  ymin=-1  ymax=1
  p : Outport  PortDimensions=3  SampleTime=0.01
      mask Display: e = 0.06;c1 = [120 230 180]/255;c2 = ([120 230 180]+0)/(256+128);c3 = ([120 230 180]+128)/(256+128);patch([0 1 1 0],[0 0 1 1],c1);patch([0 1 1 1-e 1-e 0+e],[0 0 1 1-e 0+e 0+e],c2);patch([0 0 1 1-e 0+e 0+e],[0 1 1 1-e 1-e 0+e],c3);plot([0 1 1 0 0],[0 0 1 1 0]);
  wires:
  mapminmax/1 -> p/1
  x/1 -> mapminmax/1

== system finalpro/Feed-Forward Neural Network1/Process Output 1 ==
  a : Inport  PortDimensions=1  SampleTime=0.01
      mask Display: e = 0.06;c1 = [120 230 180]/255;c2 = ([120 230 180]+0)/(256+128);c3 = ([120 230 180]+128)/(256+128);patch([0 1 1 0],[0 0 1 1],c1);patch([0 1 1 1-e 1-e 0+e],[0 0 1 1-e 0+e 0+e],c2);patch([0 0 1 1-e 0+e 0+e],[0 1 1 1-e 1-e 0+e],c3);plot([0 1 1 0 0],[0 0 1 1 0]);
  mapminmax_reverse : neural/Processing Functions/mapminmax_reverse  xmin=-289.038981665538017296057660133  xmax=289.039818879355209446657681838  ymin=-1  ymax=1
  y : Outport  PortDimensions=1  SampleTime=0.01
      mask Display: e = 0.06;c1 = [120 230 180]/255;c2 = ([120 230 180]+0)/(256+128);c3 = ([120 230 180]+128)/(256+128);patch([0 1 1 0],[0 0 1 1],c1);patch([0 1 1 1-e 1-e 0+e],[0 0 1 1-e 0+e 0+e],c2);patch([0 0 1 1-e 0+e 0+e],[0 1 1 1-e 1-e 0+e],c3);plot([0 1 1 0 0],[0 0 1 1 0]);
  wires:
  mapminmax_reverse/1 -> y/1
  a/1 -> mapminmax_reverse/1

== system finalpro/Feed-Forward Neural Network1/Layer 1/Delays 1 ==
  "p{1}" : Inport  PortDimensions=3  SampleTime=0.01
      mask Display: e = 0.06;c1 = [120 230 180]/255;c2 = ([120 230 180]+0)/(256+128);c3 = ([120 230 180]+128)/(256+128);patch([0 1 1 0],[0 0 1 1],c1);patch([0 1 1 1-e 1-e 0+e],[0 0 1 1-e 0+e 0+e],c2);patch([0 0 1 1-e 0+e 0+e],[0 1 1 1-e 1-e 0+e],c3);plot([0 1 1 0 0],[0 0 1 1 0]);
  mux : Mux  Inputs=1
      mask Display: e = 0.06;c1 = [120 150 230]/255;c2 = ([120 150 230]+0)/383;c3 = ([120 150 230]+128)/383;patch([0 1 1 0],[0 0 1 1],c1);patch([0 1 1 1-e 1-e 0+e],[0 0 1 1-e 0+e 0+e],c2);patch([0 0 1 1-e 0+e 0+e],[0 1 1 1-e 1-e 0+e],c3);plot([0 1 1 0 0],[0 0 1 1 0]);disp('Mux')
  "pd{1,1}" : Outport
      mask Display: e = 0.06;c1 = [120 230 180]/255;c2 = ([120 230 180]+0)/(256+128);c3 = ([120 230 180]+128)/(256+128);patch([0 1 1 0],[0 0 1 1],c1);patch([0 1 1 1-e 1-e 0+e],[0 0 1 1-e 0+e 0+e],c2);patch([0 0 1 1-e 0+e 0+e],[0 1 1 1-e 1-e 0+e],c3);plot([0 1 1 0 0],[0 0 1 1 0]);
  wires:
  mux/1 -> "pd{1,1}"/1
  "p{1}"/1 -> mux/1

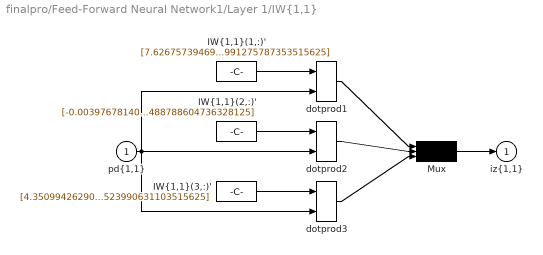
== system finalpro/Feed-Forward Neural Network1/Layer 1/IW{1,1} ==
  "pd{1,1}" : Inport  PortDimensions=3  SampleTime=0.01
      mask Display: e = 0.06;c1 = [120 230 180]/255;c2 = ([120 230 180]+0)/(256+128);c3 = ([120 230 180]+128)/(256+128);patch([0 1 1 0],[0 0 1 1],c1);patch([0 1 1 1-e 1-e 0+e],[0 0 1 1-e 0+e 0+e],c2);patch([0 0 1 1-e 0+e 0+e],[0 1 1 1-e 1-e 0+e],c3);plot([0 1 1 0 0],[0 0 1 1 0]);
  "IW{1,1}(1,:)'" : Constant  Value=[7.62675739469773628087523320573382079601287841796875;-0.5446236789066098982203811829094775021076202392578125;0.204331324162682348433150991695583797991275787353515625]
      mask Display: e = 0.06;c1 = [120 150 230]/255;c2 = ([120 150 230]+0)/383;c3 = ([120 150 230]+128)/383;patch([0 1 1 0],[0 0 1 1],c1);patch([0 1 1 1-e 1-e 0+e],[0 0 1 1-e 0+e 0+e],c2);patch([0 0 1 1-e 0+e 0+e],[0 1 1 1-e 1-e 0+e],c3);plot([0 1 1 0 0],[0 0 1 1 0]);disp('Weights');
  "IW{1,1}(2,:)'" : Constant  Value=[-0.003976781406184483162735698869028055923990905284881591796875;4.7496947825762703132568276487290859222412109375;0.003744712794989319033789332280548478593118488788604736328125]
      mask Display: e = 0.06;c1 = [120 150 230]/255;c2 = ([120 150 230]+0)/383;c3 = ([120 150 230]+128)/383;patch([0 1 1 0],[0 0 1 1],c1);patch([0 1 1 1-e 1-e 0+e],[0 0 1 1-e 0+e 0+e],c2);patch([0 0 1 1-e 0+e 0+e],[0 1 1 1-e 1-e 0+e],c3);plot([0 1 1 0 0],[0 0 1 1 0]);disp('Weights');
  "IW{1,1}(3,:)'" : Constant  Value=[4.35099426290350610457835500710643827915191650390625;-0.376883520126434390373759697467903606593608856201171875;-0.033725710150871814063666676020147860981523990631103515625]
      mask Display: e = 0.06;c1 = [120 150 230]/255;c2 = ([120 150 230]+0)/383;c3 = ([120 150 230]+128)/383;patch([0 1 1 0],[0 0 1 1],c1);patch([0 1 1 1-e 1-e 0+e],[0 0 1 1-e 0+e 0+e],c2);patch([0 0 1 1-e 0+e 0+e],[0 1 1 1-e 1-e 0+e],c3);plot([0 1 1 0 0],[0 0 1 1 0]);disp('Weights');
  Mux : Mux  Inputs=3
      mask Display: e = 0.06;c1 = [120 150 230]/255;c2 = ([120 150 230]+0)/383;c3 = ([120 150 230]+128)/383;patch([0 1 1 0],[0 0 1 1],c1);patch([0 1 1 1-e 1-e 0+e],[0 0 1 1-e 0+e 0+e],c2);patch([0 0 1 1-e 0+e 0+e],[0 1 1 1-e 1-e 0+e],c3);plot([0 1 1 0 0],[0 0 1 1 0]);disp('Mux');
  dotprod1 : neural/Weight Functions/dotprod
  dotprod2 : neural/Weight Functions/dotprod
  dotprod3 : neural/Weight Functions/dotprod
  "iz{1,1}" : Outport
      mask Display: e = 0.06;c1 = [120 230 180]/255;c2 = ([120 230 180]+0)/(256+128);c3 = ([120 230 180]+128)/(256+128);patch([0 1 1 0],[0 0 1 1],c1);patch([0 1 1 1-e 1-e 0+e],[0 0 1 1-e 0+e 0+e],c2);patch([0 0 1 1-e 0+e 0+e],[0 1 1 1-e 1-e 0+e],c3);plot([0 1 1 0 0],[0 0 1 1 0]);
  wires:
  Mux/1 -> "iz{1,1}"/1
  dotprod3/1 -> Mux/3
  "IW{1,1}(3,:)'"/1 -> dotprod3/1
  dotprod2/1 -> Mux/2
  "IW{1,1}(2,:)'"/1 -> dotprod2/1
  dotprod1/1 -> Mux/1
  "pd{1,1}"/1 -> dotprod3/2, dotprod2/2, dotprod1/2
  "IW{1,1}(1,:)'"/1 -> dotprod1/1

== system finalpro/Feed-Forward Neural Network1/Layer 2/Delays 1 ==
  "p{2}" : Inport  PortDimensions=3  SampleTime=0.01
      mask Display: e = 0.06;c1 = [120 230 180]/255;c2 = ([120 230 180]+0)/(256+128);c3 = ([120 230 180]+128)/(256+128);patch([0 1 1 0],[0 0 1 1],c1);patch([0 1 1 1-e 1-e 0+e],[0 0 1 1-e 0+e 0+e],c2);patch([0 0 1 1-e 0+e 0+e],[0 1 1 1-e 1-e 0+e],c3);plot([0 1 1 0 0],[0 0 1 1 0]);
  mux : Mux  Inputs=1
      mask Display: e = 0.06;c1 = [120 150 230]/255;c2 = ([120 150 230]+0)/383;c3 = ([120 150 230]+128)/383;patch([0 1 1 0],[0 0 1 1],c1);patch([0 1 1 1-e 1-e 0+e],[0 0 1 1-e 0+e 0+e],c2);patch([0 0 1 1-e 0+e 0+e],[0 1 1 1-e 1-e 0+e],c3);plot([0 1 1 0 0],[0 0 1 1 0]);disp('Mux')
  "pd{2,1}" : Outport
      mask Display: e = 0.06;c1 = [120 230 180]/255;c2 = ([120 230 180]+0)/(256+128);c3 = ([120 230 180]+128)/(256+128);patch([0 1 1 0],[0 0 1 1],c1);patch([0 1 1 1-e 1-e 0+e],[0 0 1 1-e 0+e 0+e],c2);patch([0 0 1 1-e 0+e 0+e],[0 1 1 1-e 1-e 0+e],c3);plot([0 1 1 0 0],[0 0 1 1 0]);
  wires:
  mux/1 -> "pd{2,1}"/1
  "p{2}"/1 -> mux/1

== system finalpro/Feed-Forward Neural Network1/Layer 2/LW{2,1} ==
  "ad{2,1}" : Inport  PortDimensions=3  SampleTime=0.01
      mask Display: e = 0.06;c1 = [120 230 180]/255;c2 = ([120 230 180]+0)/(256+128);c3 = ([120 230 180]+128)/(256+128);patch([0 1 1 0],[0 0 1 1],c1);patch([0 1 1 1-e 1-e 0+e],[0 0 1 1-e 0+e 0+e],c2);patch([0 0 1 1-e 0+e 0+e],[0 1 1 1-e 1-e 0+e],c3);plot([0 1 1 0 0],[0 0 1 1 0]);
  "IW{2,1}(1,:)'" : Constant  Value=[1.2606740079756655337206439071451313793659210205078125;0.9550747593310602301386325052590109407901763916015625;0.57590711305542263698242777536506764590740203857421875]
      mask Display: e = 0.06;c1 = [120 150 230]/255;c2 = ([120 150 230]+0)/383;c3 = ([120 150 230]+128)/383;patch([0 1 1 0],[0 0 1 1],c1);patch([0 1 1 1-e 1-e 0+e],[0 0 1 1-e 0+e 0+e],c2);patch([0 0 1 1-e 0+e 0+e],[0 1 1 1-e 1-e 0+e],c3);plot([0 1 1 0 0],[0 0 1 1 0]);disp('weights');
  Mux : Mux  Inputs=1
      mask Display: e = 0.06;c1 = [120 150 230]/255;c2 = ([120 150 230]+0)/383;c3 = ([120 150 230]+128)/383;patch([0 1 1 0],[0 0 1 1],c1);patch([0 1 1 1-e 1-e 0+e],[0 0 1 1-e 0+e 0+e],c2);patch([0 0 1 1-e 0+e 0+e],[0 1 1 1-e 1-e 0+e],c3);plot([0 1 1 0 0],[0 0 1 1 0]);disp('Mux');
  dotprod1 : neural/Weight Functions/dotprod
  "lz{2,1}" : Outport
      mask Display: e = 0.06;c1 = [120 230 180]/255;c2 = ([120 230 180]+0)/(256+128);c3 = ([120 230 180]+128)/(256+128);patch([0 1 1 0],[0 0 1 1],c1);patch([0 1 1 1-e 1-e 0+e],[0 0 1 1-e 0+e 0+e],c2);patch([0 0 1 1-e 0+e 0+e],[0 1 1 1-e 1-e 0+e],c3);plot([0 1 1 0 0],[0 0 1 1 0]);
  wires:
  Mux/1 -> "lz{2,1}"/1
  dotprod1/1 -> Mux/1
  "ad{2,1}"/1 -> dotprod1/2
  "IW{2,1}(1,:)'"/1 -> dotprod1/1
